simulink model "BestStep1"  (R2020b)
settings: Solver=ode45  StartTime=0.0  StopTime=10  RelTol=1e-3
undefined symbols (not defined in the file or in its folder): daq, degs2rpm, robust, rpm2rads, sens, ss
libraries: simulink x1
settings Model: Creator=Utente  LastModifiedBy=Utente

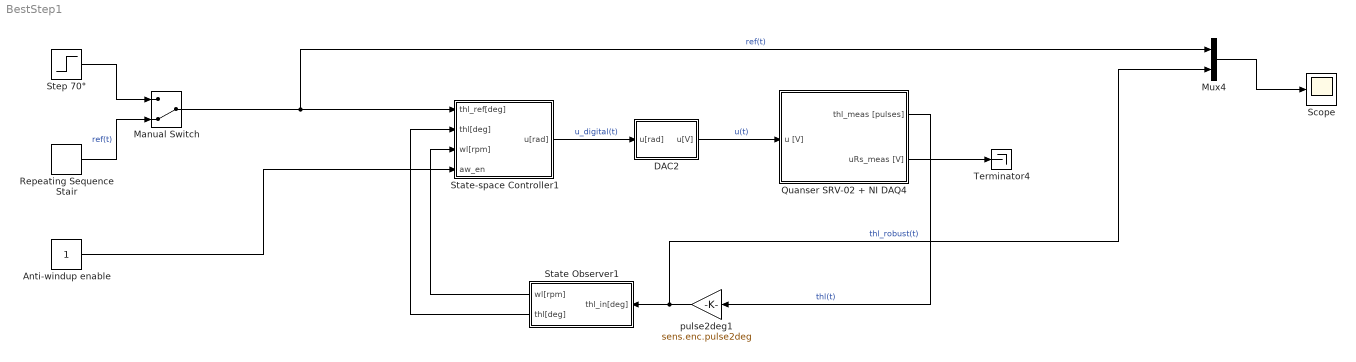
== system BestStep1 ==
  Anti-windup enable : Constant
  DAC2 : Subsystem
  Manual Switch : ManualSwitch  CurrentSetting=0
  Mux4 : Mux  Inputs=2
  Quanser SRV-02 + NI DAQ4 : Subsystem  mask(Quanser SRV-02 (with inertial load) + NI DAQ){Ts=0.001, fricType=Karnopp}
      mask prompts: Ts "NI DAQ Sample Time:"; fricType "Friction model"
      mask help: Quanser SRV-02 (with inertial load) + NI DAQ model.
      mask init:
      | %%  Sensors data
      | 
      | %   shunt resistor
      | sens.curr.Rs = 0.5;                         %   resistance [Ohm]   
      | sens.curr.uRs_std = 0.01;                   %   voltage noise standard dev [V]                           
      | sens.curr.uRs_var = sens.curr.uRs_std^2;	%   voltage noise variance [V^2]
      | 
      | %   Hewlett-Packard HEDS-5540#A06 optical encoder
      | sens.enc.ppr = 500*4;                       %   pulses per rotation
      | sens.enc.pulse2deg = 360/sens.enc.ppr;      %   [pulses] -> [deg]
      | sens.enc.pulse2rad = 2*pi/sens.enc.ppr;     %   [pulses] -> [rad]
      | sens.enc.deg2pulse = sens.enc.ppr/360;      %   [deg] -> [pulses]
      | sens.enc.rad2pulse = sens.enc.ppr/2/pi;     %   [rad] -> [pulses]
      | 
      | 
      | %%  Data acquisition board (daq) data
      | 
      | %   NI PCI-6221 DAC data
      | daq.dac.bits = 16;                                  %   resolution (bits)
      | daq.dac.fs   = 10;                                  %   full scale 
      | daq.dac.q    = 2*daq.dac.fs/(2^daq.dac.bits-1);     %	quantization
      | 
      | %   NI PCI-6221 ADC data
      | daq.adc.bits = 16;                                  %   resolution (bits)
      | daq.adc.fs   = 10;                                  %   full scale (as set in SLDRT Analog Input block)
      | daq.adc.q    = 2*daq.adc.fs/(2^daq.adc.bits-1);     %   quantization
      mask Help:
      | Riccardo Antonello (antonello@dei.unipd.it)
      | 
      | April 24, 2020
      | 
      | Dept. of Information Engineering, University of Padova
      mask TypeOptions fricType: Coulomb + viscous | Karnopp
  Repeating Sequence Stair : simulink/Sources/Repeating Sequence Stair  OutValues=[10 20 30 40 50 60 70 80 90 100].'  tsamp=1  OutMin=[]  OutMax=[]  OutDataTypeStr=double  OutputDataTypeScalingMode=double  OutDataType=fixdt(0,8)  ConRadixGroup=Best Precision: Vector-wise  OutScaling=2^-12
  Scope : Scope
  State Observer1 : Subsystem
  State-space Controller1 : Subsystem
  Step 70° : Step  Time=0  After=70  SampleTime=0
  Terminator4 : Terminator
  pulse2deg1 : Gain  Gain=sens.enc.pulse2deg
  wires:
  State-space Controller1/1(u[rad]) -> DAC2/1(u[rad])  "u_digital(t)"
  Quanser SRV-02 + NI DAQ4/1(thl_meas [pulses]) -> pulse2deg1/1  "thl(t)"
  State Observer1/2(thl[deg]) -> State-space Controller1/2(thl[deg])
  pulse2deg1/1 -> Mux4/2, State Observer1/1(thl_in[deg])  "thl_robust(t)"
  State Observer1/1(wl[rpm]) -> State-space Controller1/3(wl[rpm])
  Anti-windup enable/1 -> State-space Controller1/4(aw_en)
  DAC2/1(u[V]) -> Quanser SRV-02 + NI DAQ4/1(u [V])  "u(t)"
  Quanser SRV-02 + NI DAQ4/2(uRs_meas [V]) -> Terminator4/1
  Mux4/1 -> Scope/1
  Manual Switch/1 -> State-space Controller1/1(thl_ref[deg]), Mux4/1  "ref(t)"
  Repeating Sequence Stair/1 -> Manual Switch/2  "ref(t)"
  Step 70°/1 -> Manual Switch/1

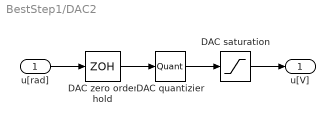
== system BestStep1/DAC2 ==
  u[rad] : Inport
  DAC quantizier : Quantizer  QuantizationInterval=daq.dac.q
  DAC saturation : Saturate  UpperLimit=daq.dac.vdd  LowerLimit=daq.dac.vss
  DAC zero order hold : ZeroOrderHold  SampleTime=daq.dac.T_s
  u[V] : Outport
  wires:
  DAC quantizier/1 -> DAC saturation/1
  DAC zero order hold/1 -> DAC quantizier/1
  DAC saturation/1 -> u[V]/1
  u[rad]/1 -> DAC zero order hold/1

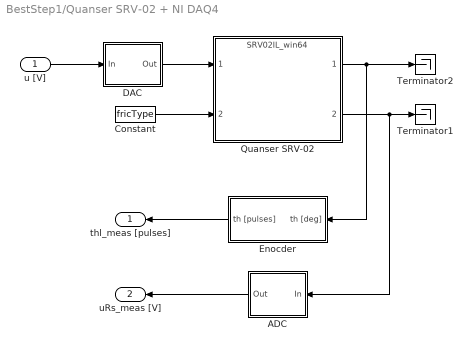
== system BestStep1/Quanser SRV-02 + NI DAQ4 ==
  u [V] : Inport
  ADC : Subsystem
  Constant : Constant  Value=fricType
  DAC : Subsystem
  Enocder : Subsystem
  Quanser SRV-02 : ModelReference  ModelNameDialog=SRV02IL_win64.slxp  ModelReferenceVersion=1.44  CopyOfModelProtected=on
  Terminator1 : Terminator
  Terminator2 : Terminator
  thl_meas [pulses] : Outport
  uRs_meas [V] : Outport  Port=2
  wires:
  Enocder/1(th [pulses]) -> thl_meas [pulses]/1
  ADC/1(Out) -> uRs_meas [V]/1
  DAC/1(Out) -> Quanser SRV-02/1
  Quanser SRV-02/2 -> ADC/1(In), Terminator1/1
  u [V]/1 -> DAC/1(In)
  Quanser SRV-02/1 -> Enocder/1(th [deg]), Terminator2/1
  Constant/1 -> Quanser SRV-02/2

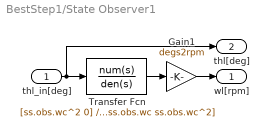
== system BestStep1/State Observer1 ==
  thl_in[deg] : Inport
  Gain1 : Gain  Gain=degs2rpm
  Transfer Fcn : TransferFcn  Numerator=[ss.obs.wc^2 0]  Denominator=[1 2*ss.obs.delta*ss.obs.wc ss.obs.wc^2]
  wl[rpm] : Outport
  thl[deg] : Outport  Port=2
  wires:
  Transfer Fcn/1 -> Gain1/1
  thl_in[deg]/1 -> thl[deg]/1, Transfer Fcn/1
  Gain1/1 -> wl[rpm]/1

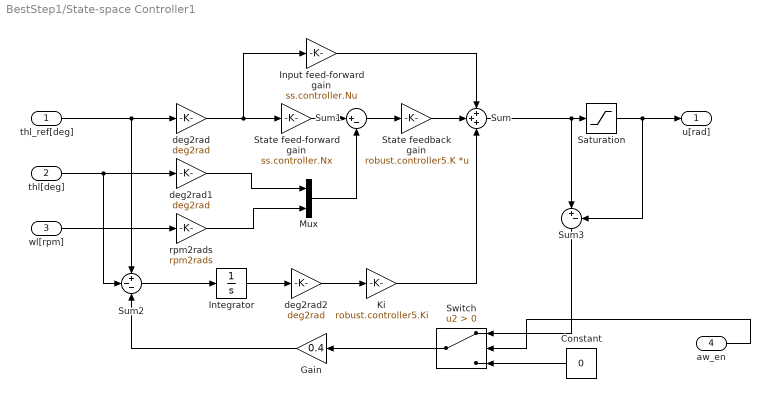
== system BestStep1/State-space Controller1 ==
  thl_ref[deg] : Inport
  thl[deg] : Inport  Port=2
  wl[rpm] : Inport  Port=3
  aw_en : Inport  Port=4
  Constant : Constant  Value=0
  Gain : Gain  Gain=0.4
  Input feed-forward gain : Gain  Gain=ss.controller.Nu
  Integrator : Integrator
  Ki : Gain  Gain=robust.controller5.Ki
  Mux : Mux  Inputs=2
  Saturation : Saturate  UpperLimit=daq.dac.vdd  LowerLimit=daq.dac.vss
  State feed-forward gain : Gain  Gain=ss.controller.Nx
  State feedback gain : Gain  Gain=robust.controller5.K  Multiplication=Matrix(K*u)
  Sum : Sum  Inputs=+++
  Sum1 : Sum  Inputs=|+-
  Sum2 : Sum  Inputs=+--
  Sum3 : Sum  Inputs=|+-
  Switch : Switch  Criteria=u2 > Threshold
  deg2rad : Gain  Gain=deg2rad
  deg2rad1 : Gain  Gain=deg2rad
  deg2rad2 : Gain  Gain=deg2rad
  rpm2rads : Gain  Gain=rpm2rads
  u[rad] : Outport
  wires:
  rpm2rads/1 -> Mux/2
  Sum1/1 -> State feedback gain/1
  Mux/1 -> Sum1/2
  thl_ref[deg]/1 -> Sum2/1, deg2rad/1
  deg2rad/1 -> Input feed-forward gain/1, State feed-forward gain/1
  State feed-forward gain/1 -> Sum1/1
  deg2rad1/1 -> Mux/1
  Saturation/1 -> Sum3/2, u[rad]/1
  wl[rpm]/1 -> rpm2rads/1
  thl[deg]/1 -> Sum2/2, deg2rad1/1
  State feedback gain/1 -> Sum/2
  Sum/1 -> Sum3/1, Saturation/1
  Sum2/1 -> Integrator/1
  Integrator/1 -> deg2rad2/1
  deg2rad2/1 -> Ki/1
  Ki/1 -> Sum/3
  Gain/1 -> Sum2/3
  Switch/1 -> Gain/1
  Sum3/1 -> Switch/1
  Constant/1 -> Switch/3
  aw_en/1 -> Switch/2
  Input feed-forward gain/1 -> Sum/1

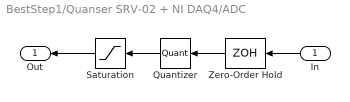
== system BestStep1/Quanser SRV-02 + NI DAQ4/ADC ==
  In : Inport
  Quantizer : Quantizer  QuantizationInterval=daq.adc.q
  Saturation : Saturate  UpperLimit=daq.adc.fs  LowerLimit=-daq.adc.fs
  Zero-Order Hold : ZeroOrderHold  SampleTime=Ts
  Out : Outport
  wires:
  Saturation/1 -> Out/1
  In/1 -> Zero-Order Hold/1
  Quantizer/1 -> Saturation/1
  Zero-Order Hold/1 -> Quantizer/1

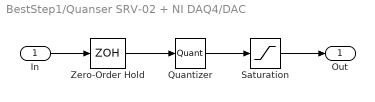
== system BestStep1/Quanser SRV-02 + NI DAQ4/DAC ==
  In : Inport
  Quantizer : Quantizer  QuantizationInterval=daq.dac.q
  Saturation : Saturate  UpperLimit=daq.dac.fs  LowerLimit=-daq.dac.fs
  Zero-Order Hold : ZeroOrderHold  SampleTime=Ts
  Out : Outport
  wires:
  Quantizer/1 -> Saturation/1
  In/1 -> Zero-Order Hold/1
  Zero-Order Hold/1 -> Quantizer/1
  Saturation/1 -> Out/1

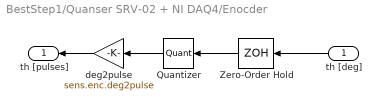
== system BestStep1/Quanser SRV-02 + NI DAQ4/Enocder ==
  th [deg] : Inport
  Quantizer : Quantizer  QuantizationInterval=sens.enc.pulse2deg
  Zero-Order Hold : ZeroOrderHold  SampleTime=Ts
  deg2pulse : Gain  Gain=sens.enc.deg2pulse
  th [pulses] : Outport
  wires:
  Quantizer/1 -> deg2pulse/1
  th [deg]/1 -> Zero-Order Hold/1
  Zero-Order Hold/1 -> Quantizer/1
  deg2pulse/1 -> th [pulses]/1
